simulink library "Ta_Library"  (R2019b)
settings: Solver=VariableStepAuto  StartTime=0.0  StopTime=10.0  RelTol=1e-3
undefined symbols (not defined in the file): AEBSFunctionLib, StateDelayAbortion, TargetClassification
libraries: Mylibrary x5, simulink x1
(part 1 of 3)
settings Model: Creator=hezhaoyang  LastModifiedBy=86156

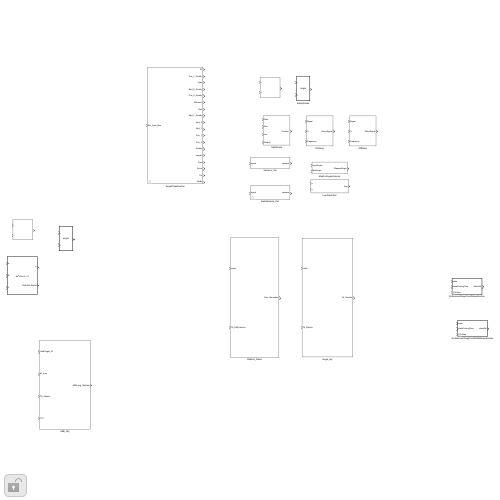
[thumbnail: Simulink's stored preview of the top-level diagram]
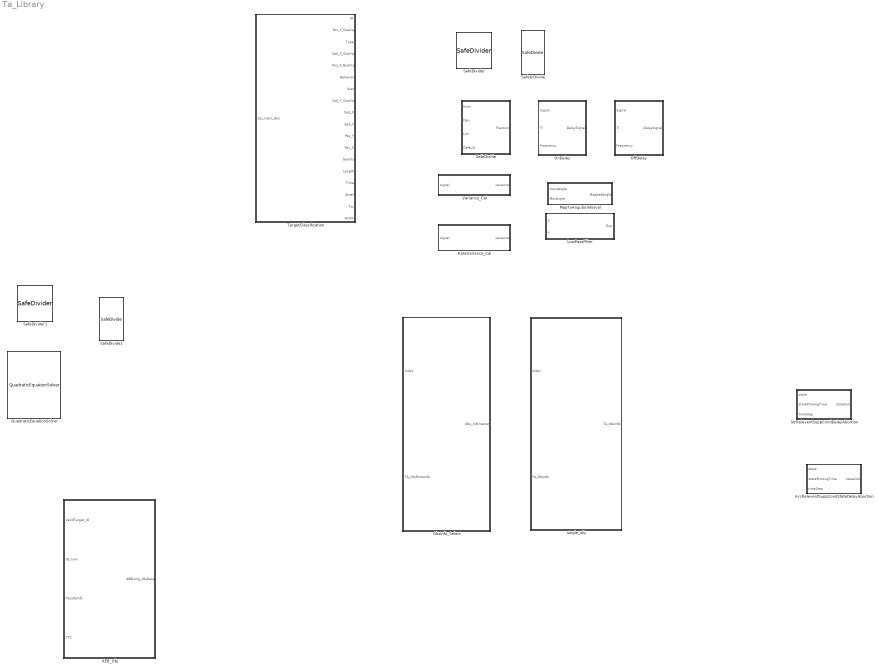
== system Ta_Library ==
  AEB_Obj : Subsystem
  AccReleventSuppCondStateDelayAbortion : Subsystem  AncestorBlock=AEBSFunctionLib/StateDelayAbortion  TreatAsAtomicUnit=on
  LowPassFilter : Subsystem
  MapToAngularInterval : Subsystem
  ObsInfo_Select : Subsystem
  OffDelay : Subsystem
  OnDelay : Subsystem
  QuadraticEquationSolver : Mylibrary/QuadraticEquationSolver  ZeroThreshold=single(1e-2)
  RateVariance_Cal : Subsystem  AncestorBlock=Ta_Library/Variance_Cal
  SafeDivide : Subsystem
  SafeDivide1 : Mylibrary/SafeDivide  DataType=single  DataTypeMax=0  DataTypeMin=0
  SafeDivider : Mylibrary/SafeDivider  SystemSampleTime=-1  Latency=0  AutoFrameSizeCalculation=off
  SafeDivider1 : Mylibrary/SafeDivider  SystemSampleTime=-1  Latency=0  AutoFrameSizeCalculation=off
  SafetyDivide : Mylibrary/SafeDivide  DataType=single  DataTypeMax=0  DataTypeMin=0
  StrReleventSuppCondDelayAbortion : Subsystem  AncestorBlock=AEBSFunctionLib/StateDelayAbortion  TreatAsAtomicUnit=on
  TargetClassification : Subsystem  AncestorBlock=TargetClassification/TargetClassification
  Variance_Cal : Subsystem
  single_obj : Subsystem

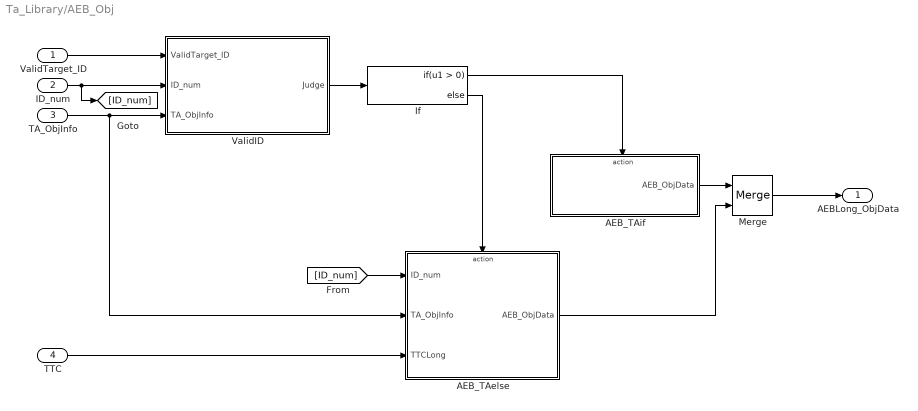
== system Ta_Library/AEB_Obj ==
  ValidTarget_ID : Inport
  ID_num : Inport  Port=2
  TA_ObjInfo : Inport  Port=3
  TTC : Inport  Port=4
  AEB_TAelse : Subsystem  TreatAsAtomicUnit=on
  AEB_TAif : Subsystem  TreatAsAtomicUnit=on
  If : If
  Merge : Merge
  ValidID : Subsystem
  AEBLong_ObjData : Outport
  wires:
  ValidID/1(Judge) -> If/1
  If/1 -> AEB_TAif/Action
  TA_ObjInfo/1 -> AEB_TAelse/2(TA_ObjInfo), ValidID/3(TA_ObjInfo)
  If/2 -> AEB_TAelse/Action
  ID_num/1 -> [ID_num], ValidID/2(ID_num)
  AEB_TAif/1(AEB_ObjData) -> Merge/1
  AEB_TAelse/1(AEB_ObjData) -> Merge/2
  Merge/1 -> AEBLong_ObjData/1
  ValidTarget_ID/1 -> ValidID/1(ValidTarget_ID)
  [ID_num] -> AEB_TAelse/1(ID_num)
  TTC/1 -> AEB_TAelse/3(TTCLong)

== system Ta_Library/AccReleventSuppCondStateDelayAbortion ==
  state : Inport
  stateProlongTime : Inport  Port=2
  timeStep : Inport  Port=3
  StateDelayAbortion : Stateflow chart  TreatAsAtomicUnit=on
  Terminator : Terminator
  Unit Delay : UnitDelay  SampleTime=-1  HasFrameUpgradeWarning=on
  stateOut : Outport
  wires:
  state/1 -> Unit Delay/1, StateDelayAbortion/1(state)
  Unit Delay/1 -> StateDelayAbortion/2(stateK1)
  stateProlongTime/1 -> StateDelayAbortion/3(stateProlongationTime)
  timeStep/1 -> StateDelayAbortion/4(Ts)
  StateDelayAbortion/1(timeSinceLastState) -> Terminator/1
  StateDelayAbortion/2(stateOut) -> stateOut/1

== system Ta_Library/LowPassFilter ==
  a : Inport
  u : Inport  Port=2
  Add3 : Sum
  Delay1 : Delay  DelayLength=1
  Product1 : Product
  Subtract : Sum  Inputs=+-
  Exp : Outport  VectorParamsAs1DForOutWhenUnconnected=off
  wires:
  a/1 -> Product1/1
  Add3/1 -> Delay1/1, Exp/1
  Product1/1 -> Add3/1
  Delay1/1 -> Subtract/2, Add3/2
  Subtract/1 -> Product1/2
  u/1 -> Subtract/1

== system Ta_Library/MapToAngularInterval ==
  note: Map the input angle to an interval between [-MaxAngle, MaxAngle].
  InputAngle : Inport
  MaxAngle : Inport  Port=2
  Gain_1 : Gain  Gain=2  OutDataTypeStr=single
  Modulus : Math  Operator=mod  SignedPower=on  SaturateOnIntegerOverflow=on
  Subtract_1 : Sum  Inputs=-+  OutDataTypeStr=single
  Subtract_2 : Sum  Inputs=+-  OutDataTypeStr=single
  MappedAngle : Outport
  wires:
  [MaxAngle] -> Subtract_2/1
  Gain_1/1 -> Modulus/2
  MaxAngle/1 -> [MaxAngle], Subtract_1/2, Gain_1/1  "MaxAngle"
  InputAngle/1 -> Subtract_1/1  "InputAngle"
  Subtract_1/1 -> Modulus/1
  Modulus/1 -> Subtract_2/2
  Subtract_2/1 -> MappedAngle/1  "MappedAngle"

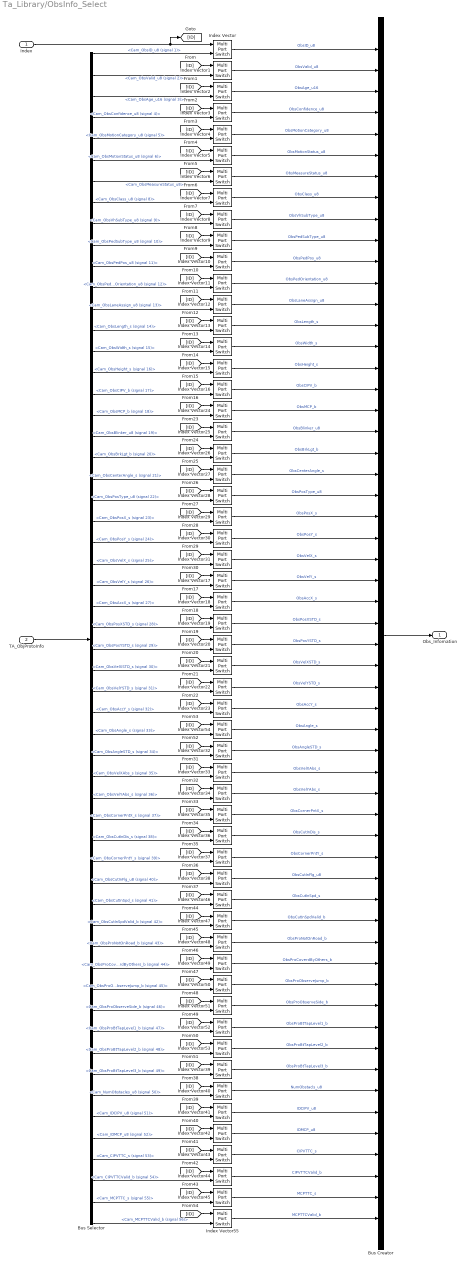
== system Ta_Library/ObsInfo_Select ==
  Index : Inport
  TA_ObjProtoInfo : Inport  Port=2
  Bus Creator : BusCreator  Inputs=56
  Bus Selector : BusSelector  OutputSignals=Cam_ObsID_u8 (signal 1),Cam_ObsValid_u8 (signal 2),Cam_ObsAge_u16 (signal 3),Cam_ObsConfidence_u8 (signal 4),Cam_ObsMotionCategory_u8 (signal 5),Cam_ObsMotionStatus_u8 (signal 6),Cam_ObsMeasureStatus_u8,Cam_ObsClass_u8 (signal 8),Cam_ObsVhSubType_u8 (signal 9),Cam_ObsPedSubType_u8 (signal 10),Cam_ObsPedPos_u8 (signal 11),Cam_ObsPedOrientation_u8 (signal 12),Cam_ObsLaneAssign_u8 (signal 13),Cam_ObsLength_s (signal 14),Cam_ObsWidth_s (signal 15),Cam_ObsHeight_s (signal 16),Cam_ObsCIPV_b (signal 17),Cam_ObsMCP_b (signal 18),Cam_ObsBlinker_u8 (signal 19),Cam_ObsBrkLgt_b (signal 20),Cam_ObsCenterAngle_s (signal 21),Cam_ObsPosType_u8 (signal 22),Cam_ObsPosX_s (signal 23),Cam_ObsPosY_s (signal 24),Cam_ObsVelX_s (signal 25),Cam_ObsVelY_s (signal 26),Cam_ObsAccX_s (signal 27),Cam_ObsPosXSTD_s (signal 28),Cam_ObsPosYSTD_s (signal 29),Cam_ObsVelXSTD_s (signal 30),Cam_ObsVelYSTD_s (signal 31),Cam_ObsAccY_s (signal 32),Cam_ObsAngle_s (signal 33),Cam_ObsAngleSTD_s (signal 34),Cam_ObsVelXAbs_s (signal 35),Cam_ObsVelYAbs_s (signal 36),Cam_ObsCornerPntX_s (signal 37),Cam_ObsCutInDis_s (signal 38),Cam_ObsCornerPntY_s (signal 39),Cam_ObsCutInFlg_u8 (signal 40),Cam_ObsCutInSpd_s (signal 41),Cam_ObsCutInSpdValid_b (signal 42),Cam_ObsProNotOnRoad_b (signal 43),Cam_ObsProCoverdByOthers_b (signal 44),Cam_ObsProObserveJump_b (signal 45),Cam_ObsProObserveSide_b (signal 46),Cam_ObsProBtTapLevel1_b (signal 47),Cam_ObsProBtTapLevel2_b (signal 48),Cam_ObsProBtTapLevel3_b (signal 49),Cam_NumObstacles_u8 (signal 50),Cam_IDCIPV_u8 (signal 51),Cam_IDMCP_u8 (signal 52),Cam_CIPVTTC_s (signal 53),Cam_CIPVTTCValid_b (signal 54),Cam_MCPTTC_s (signal 55),Cam_MCPTTCValid_b (signal 56)
  Index Vector{,1..55} (56 alike) : MultiPortSwitch  Inputs=1
  Obs_Infomation : Outport
  wires:
  TA_ObjProtoInfo/1 -> Bus Selector/1
  Bus Selector/1 -> Index Vector/2  "<Cam_ObsID_u8 (signal 1)>"
  Index/1 -> [ID], Index Vector/1
  [ID] -> Index Vector1/1
  Bus Selector/2 -> Index Vector1/2  "<Cam_ObsValid_u8 (signal 2)>"
  Bus Selector/3 -> Index Vector2/2  "<Cam_ObsAge_u16 (signal 3)>"
  [ID] -> Index Vector2/1
  [ID] -> Index Vector4/1
  Bus Selector/5 -> Index Vector4/2  "<Cam_ObsMotionCategory_u8 (signal 5)>"
  Bus Selector/4 -> Index Vector3/2  "<Cam_ObsConfidence_u8 (signal 4)>"
  [ID] -> Index Vector3/1
  [ID] -> Index Vector7/1
  Bus Selector/8 -> Index Vector7/2  "<Cam_ObsClass_u8 (signal 8)>"
  Bus Selector/9 -> Index Vector8/2  "<Cam_ObsVhSubType_u8 (signal 9)>"
  [ID] -> Index Vector8/1
  [ID] -> Index Vector6/1
  Bus Selector/7 -> Index Vector6/2  "<Cam_ObsMeasureStatus_u8>"
  Bus Selector/6 -> Index Vector5/2  "<Cam_ObsMotionStatus_u8 (signal 6)>"
  [ID] -> Index Vector5/1
  [ID] -> Index Vector13/1
  Bus Selector/14 -> Index Vector13/2  "<Cam_ObsLength_s (signal 14)>"
  Bus Selector/15 -> Index Vector14/2  "<Cam_ObsWidth_s (signal 15)>"
  [ID] -> Index Vector14/1
  [ID] -> Index Vector16/1
  Bus Selector/16 -> Index Vector15/2  "<Cam_ObsHeight_s (signal 16)>"
  [ID] -> Index Vector15/1
  [ID] -> Index Vector11/1
  Bus Selector/12 -> Index Vector11/2  "<Cam_ObsPedOrientation_u8 (signal 12)>"
  Bus Selector/13 -> Index Vector12/2  "<Cam_ObsLaneAssign_u8 (signal 13)>"
  [ID] -> Index Vector12/1
  [ID] -> Index Vector10/1
  Bus Selector/11 -> Index Vector10/2  "<Cam_ObsPedPos_u8 (signal 11)>"
  Bus Selector/10 -> Index Vector9/2  "<Cam_ObsPedSubType_u8 (signal 10)>"
  [ID] -> Index Vector9/1
  Bus Selector/17 -> Index Vector16/2  "<Cam_ObsCIPV_b (signal 17)>"
  Bus Selector/32 -> Index Vector23/2  "<Cam_ObsAccY_s (signal 32)>"
  [ID] -> Index Vector31/1
  Bus Selector/25 -> Index Vector31/2  "<Cam_ObsVelX_s (signal 25)>"
  Bus Selector/26 -> Index Vector17/2  "<Cam_ObsVelY_s (signal 26)>"
  [ID] -> Index Vector17/1
  [ID] -> Index Vector19/1
  Bus Selector/28 -> Index Vector19/2  "<Cam_ObsPosXSTD_s (signal 28)>"
  Bus Selector/27 -> Index Vector18/2  "<Cam_ObsAccX_s (signal 27)>"
  [ID] -> Index Vector18/1
  [ID] -> Index Vector22/1
  Bus Selector/31 -> Index Vector22/2  "<Cam_ObsVelYSTD_s (signal 31)>"
  [ID] -> Index Vector23/1
  [ID] -> Index Vector21/1
  Bus Selector/30 -> Index Vector21/2  "<Cam_ObsVelXSTD_s (signal 30)>"
  Bus Selector/29 -> Index Vector20/2  "<Cam_ObsPosYSTD_s (signal 29)>"
  [ID] -> Index Vector20/1
  [ID] -> Index Vector27/1
  Bus Selector/21 -> Index Vector27/2  "<Cam_ObsCenterAngle_s (signal 21)>"
  Bus Selector/22 -> Index Vector28/2  "<Cam_ObsPosType_u8 (signal 22)>"
  [ID] -> Index Vector28/1
  [ID] -> Index Vector30/1
  Bus Selector/24 -> Index Vector30/2  "<Cam_ObsPosY_s (signal 24)>"
  Bus Selector/23 -> Index Vector29/2  "<Cam_ObsPosX_s (signal 23)>"
  [ID] -> Index Vector29/1
  [ID] -> Index Vector25/1
  Bus Selector/19 -> Index Vector25/2  "<Cam_ObsBlinker_u8 (signal 19)>"
  Bus Selector/20 -> Index Vector26/2  "<Cam_ObsBrkLgt_b (signal 20)>"
  [ID] -> Index Vector26/1
  [ID] -> Index Vector24/1
  Bus Selector/18 -> Index Vector24/2  "<Cam_ObsMCP_b (signal 18)>"
  Bus Selector/41 -> Index Vector46/2  "<Cam_ObsCutInSpd_s (signal 41)>"
  [ID] -> Index Vector46/1
  [ID] -> Index Vector48/1
  Bus Selector/43 -> Index Vector48/2  "<Cam_ObsProNotOnRoad_b (signal 43)>"
  Bus Selector/42 -> Index Vector47/2  "<Cam_ObsCutInSpdValid_b (signal 42)>"
  [ID] -> Index Vector47/1
  [ID] -> Index Vector51/1
  Bus Selector/46 -> Index Vector51/2  "<Cam_ObsProObserveSide_b (signal 46)>"
  Bus Selector/47 -> Index Vector52/2  "<Cam_ObsProBtTapLevel1_b (signal 47)>"
  [ID] -> Index Vector52/1
  [ID] -> Index Vector50/1
  Bus Selector/45 -> Index Vector50/2  "<Cam_ObsProObserveJump_b (signal 45)>"
  Bus Selector/44 -> Index Vector49/2  "<Cam_ObsProCoverdByOthers_b (signal 44)>"
  [ID] -> Index Vector49/1
  [ID] -> Index Vector42/1
  Bus Selector/52 -> Index Vector42/2  "<Cam_IDMCP_u8 (signal 52)>"
  Bus Selector/53 -> Index Vector43/2  "<Cam_CIPVTTC_s (signal 53)>"
  [ID] -> Index Vector43/1
  [ID] -> Index Vector45/1
  Bus Selector/54 -> Index Vector44/2  "<Cam_CIPVTTCValid_b (signal 54)>"
  [ID] -> Index Vector44/1
  [ID] -> Index Vector40/1
  Bus Selector/50 -> Index Vector40/2  "<Cam_NumObstacles_u8 (signal 50)>"
  Bus Selector/51 -> Index Vector41/2  "<Cam_IDCIPV_u8 (signal 51)>"
  [ID] -> Index Vector41/1
  [ID] -> Index Vector39/1
  Bus Selector/49 -> Index Vector39/2  "<Cam_ObsProBtTapLevel3_b (signal 49)>"
  Bus Selector/48 -> Index Vector53/2  "<Cam_ObsProBtTapLevel2_b (signal 48)>"
  [ID] -> Index Vector53/1
  Bus Selector/55 -> Index Vector45/2  "<Cam_MCPTTC_s (signal 55)>"
  Bus Selector/40 -> Index Vector38/2  "<Cam_ObsCutInFlg_u8 (signal 40)>"
  Bus Selector/33 -> Index Vector54/2  "<Cam_ObsAngle_s (signal 33)>"
  Bus Selector/34 -> Index Vector32/2  "<Cam_ObsAngleSTD_s (signal 34)>"
  [ID] -> Index Vector32/1
  [ID] -> Index Vector34/1
  Bus Selector/36 -> Index Vector34/2  "<Cam_ObsVelYAbs_s (signal 36)>"
  Bus Selector/35 -> Index Vector33/2  "<Cam_ObsVelXAbs_s (signal 35)>"
  [ID] -> Index Vector33/1
  [ID] -> Index Vector37/1
  Bus Selector/39 -> Index Vector37/2  "<Cam_ObsCornerPntY_s (signal 39)>"
  [ID] -> Index Vector38/1
  [ID] -> Index Vector36/1
  Bus Selector/38 -> Index Vector36/2  "<Cam_ObsCutInDis_s (signal 38)>"
  Bus Selector/37 -> Index Vector35/2  "<Cam_ObsCornerPntX_s (signal 37)>"
  [ID] -> Index Vector35/1
  [ID] -> Index Vector54/1
  Bus Selector/56 -> Index Vector55/2  "<Cam_MCPTTCValid_b (signal 56)>"
  [ID] -> Index Vector55/1
  Index Vector32/1 -> Bus Creator/34  "ObsAngleSTD_s"
  Index Vector33/1 -> Bus Creator/35  "ObsVelXAbs_s"
  Index Vector54/1 -> Bus Creator/33  "ObsAngle_s"
  Index Vector34/1 -> Bus Creator/36  "ObsVelYAbs_s"
  Index Vector23/1 -> Bus Creator/32  "ObsAccY_s"
  Index Vector35/1 -> Bus Creator/37  "ObsCornerPntX_s"
  Index Vector22/1 -> Bus Creator/31  "ObsVelYSTD_s"
  Index Vector36/1 -> Bus Creator/38  "ObsCutInDis_s"
  Index Vector21/1 -> Bus Creator/30  "ObsVelXSTD_s"
  Index Vector37/1 -> Bus Creator/39  "ObsCornerPntY_s"
  Index Vector20/1 -> Bus Creator/29  "ObsPosYSTD_s"
  Index Vector38/1 -> Bus Creator/40  "ObsCutInFlg_u8"
  Index Vector19/1 -> Bus Creator/28  "ObsPosXSTD_s"
  Index Vector46/1 -> Bus Creator/41  "ObsCutInSpd_s"
  Index Vector18/1 -> Bus Creator/27  "ObsAccX_s"
  Index Vector47/1 -> Bus Creator/42  "ObsCutInSpdValid_b"
  Index Vector17/1 -> Bus Creator/26  "ObsVelY_s"
  Index Vector48/1 -> Bus Creator/43  "ObsProNotOnRoad_b"
  Index Vector31/1 -> Bus Creator/25  "ObsVelX_s"
  Index Vector49/1 -> Bus Creator/44  "ObsProCoverdByOthers_b"
  Index Vector30/1 -> Bus Creator/24  "ObsPosY_s"
  Index Vector50/1 -> Bus Creator/45  "ObsProObserveJump_b"
  Index Vector29/1 -> Bus Creator/23  "ObsPosX_s"
  Index Vector51/1 -> Bus Creator/46  "ObsProObserveSide_b"
  Index Vector28/1 -> Bus Creator/22  "ObsPosType_u8"
  Index Vector52/1 -> Bus Creator/47  "ObsProBtTapLevel1_b"
  Index Vector27/1 -> Bus Creator/21  "ObsCenterAngle_s"
  Index Vector53/1 -> Bus Creator/48  "ObsProBtTapLevel2_b"
  Index Vector26/1 -> Bus Creator/20  "ObsBrkLgt_b"
  Index Vector39/1 -> Bus Creator/49  "ObsProBtTapLevel3_b"
  Index Vector25/1 -> Bus Creator/19  "ObsBlinker_u8"
  Index Vector40/1 -> Bus Creator/50  "NumObstacls_u8"
  Index Vector24/1 -> Bus Creator/18  "ObsMCP_b"
  Index Vector41/1 -> Bus Creator/51  "IDCIPV_u8"
  Index Vector16/1 -> Bus Creator/17  "ObsCIPV_b"
  Index Vector42/1 -> Bus Creator/52  "IDMCP_u8"
  Index Vector15/1 -> Bus Creator/16  "ObsHeight_s"
  Index Vector43/1 -> Bus Creator/53  "CIPVTTC_s"
  Index Vector14/1 -> Bus Creator/15  "ObsWidth_s"
  Index Vector44/1 -> Bus Creator/54  "CIPVTTCValid_b"
  Index Vector13/1 -> Bus Creator/14  "ObsLength_s"
  Index Vector45/1 -> Bus Creator/55  "MCPTTC_s"
  Index Vector12/1 -> Bus Creator/13  "ObsLaneAssign_u8"
  Index Vector55/1 -> Bus Creator/56  "MCPTTCValid_b"
  Index Vector11/1 -> Bus Creator/12  "ObsPedOrientation_u8"
  Index Vector10/1 -> Bus Creator/11  "ObsPedPos_u8"
  Index Vector9/1 -> Bus Creator/10  "ObsPedSubType_u8"
  Index Vector8/1 -> Bus Creator/9  "ObsVhSubType_u8"
  Index Vector7/1 -> Bus Creator/8  "ObsClass_u8"
  Index Vector6/1 -> Bus Creator/7  "ObsMeasureStatus_u8"
  Index Vector5/1 -> Bus Creator/6  "ObsMotionStatus_u8"
  Index Vector4/1 -> Bus Creator/5  "ObsMotionCategory_u8"
  Index Vector3/1 -> Bus Creator/4  "ObsConfidence_u8"
  Index Vector2/1 -> Bus Creator/3  "ObsAge_u16"
  Index Vector1/1 -> Bus Creator/2  "ObsValid_u8"
  Index Vector/1 -> Bus Creator/1  "ObsID_u8"
  Bus Creator/1 -> Obs_Infomation/1

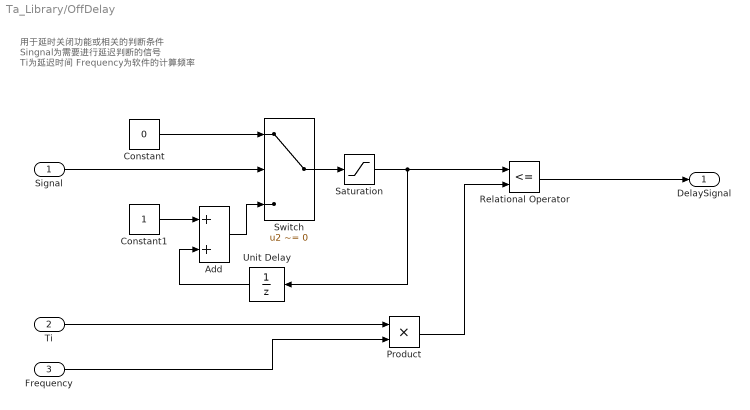
== system Ta_Library/OffDelay ==
  note: 用于延时关闭功能或相关的判断条件
      | Singnal为需要进行延迟判断的信号
      | Ti为延迟时间
      | Frequency为软件的计算频率
  Signal : Inport
  Ti : Inport  Port=2
  Frequency : Inport  Port=3
  Add : Sum
  Constant : Constant  Value=0  OutDataTypeStr=single
  Constant1 : Constant  OutDataTypeStr=single
  Product : Product
  Relational Operator : RelationalOperator  Operator=<=  OutDataTypeStr=boolean  RndMeth=Simplest
  Saturation : Saturate  UpperLimit=1000  LowerLimit=0
  Switch : Switch  Criteria=u2 ~= 0
  Unit Delay : UnitDelay  SampleTime=-1  HasFrameUpgradeWarning=on
  DelaySignal : Outport
  wires:
  Signal/1 -> Switch/2
  Ti/1 -> Product/1
  Constant1/1 -> Add/1
  Unit Delay/1 -> Add/2
  Switch/1 -> Saturation/1
  Constant/1 -> Switch/1
  Relational Operator/1 -> DelaySignal/1
  Frequency/1 -> Product/2
  Product/1 -> Relational Operator/2
  Add/1 -> Switch/3
  Saturation/1 -> Relational Operator/1, Unit Delay/1

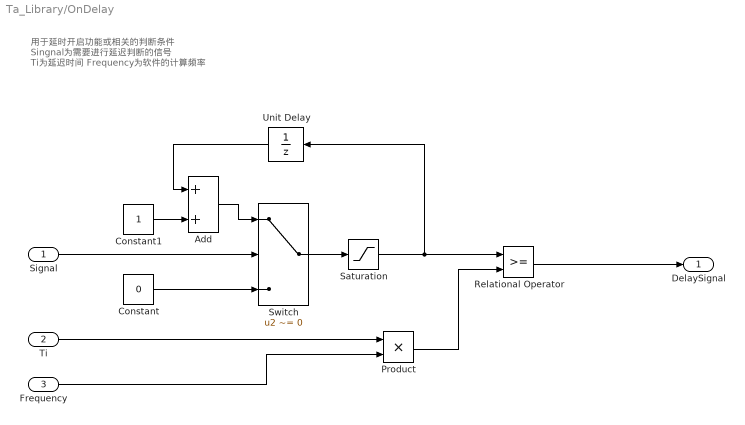
== system Ta_Library/OnDelay ==
  note: 用于延时开启功能或相关的判断条件
      | Singnal为需要进行延迟判断的信号
      | Ti为延迟时间
      | Frequency为软件的计算频率
  Signal : Inport
  Ti : Inport  Port=2
  Frequency : Inport  Port=3
  Add : Sum
  Constant : Constant  Value=0  OutDataTypeStr=single
  Constant1 : Constant  OutDataTypeStr=single
  Product : Product
  Relational Operator : RelationalOperator  OutDataTypeStr=boolean  RndMeth=Simplest
  Saturation : Saturate  UpperLimit=1000  LowerLimit=0
  Switch : Switch  Criteria=u2 ~= 0
  Unit Delay : UnitDelay  SampleTime=-1  HasFrameUpgradeWarning=on
  DelaySignal : Outport
  wires:
  Product/1 -> Relational Operator/2
  Switch/1 -> Saturation/1
  Ti/1 -> Product/1
  Signal/1 -> Switch/2
  Relational Operator/1 -> DelaySignal/1
  Frequency/1 -> Product/2
  Add/1 -> Switch/1
  Constant/1 -> Switch/3
  Constant1/1 -> Add/2
  Unit Delay/1 -> Add/1
  Saturation/1 -> Relational Operator/1, Unit Delay/1

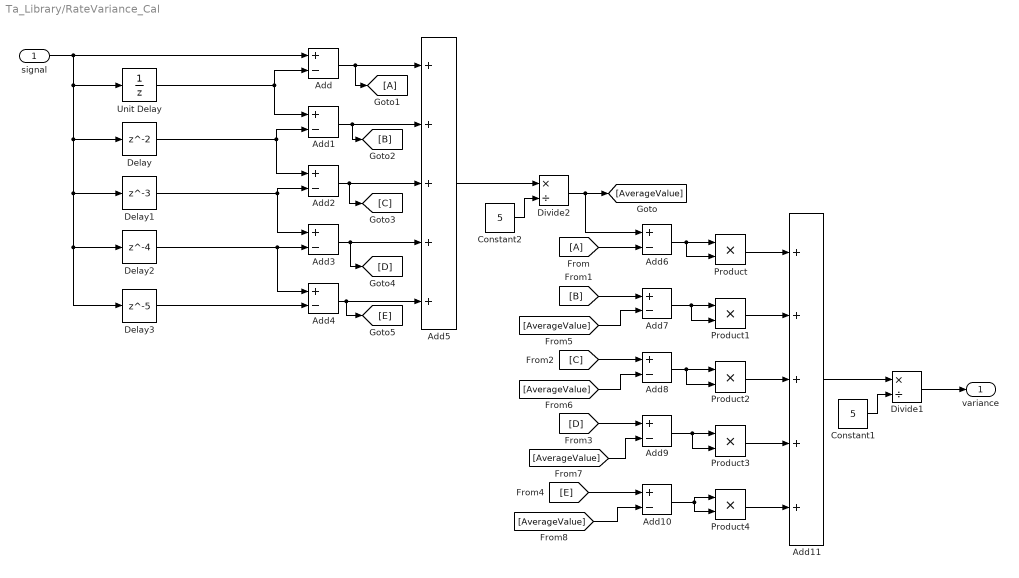
== system Ta_Library/RateVariance_Cal ==
  signal : Inport
  Add{,1..4,6..10} (10 alike) : Sum  Inputs=+-
  Add11 : Sum  Inputs=+++++
  Add5 : Sum  Inputs=+++++
  Constant1 : Constant  Value=5  OutDataTypeStr=single
  Constant2 : Constant  Value=5  OutDataTypeStr=single
  Delay : Delay
  Delay1 : Delay  DelayLength=3
  Delay2 : Delay  DelayLength=4
  Delay3 : Delay  DelayLength=5
  Divide1 : Product  Inputs=*/
  Divide2 : Product  Inputs=*/
  Product{,1..4} (5 alike) : Product
  Unit Delay : UnitDelay  SampleTime=-1  HasFrameUpgradeWarning=on
  variance : Outport
  wires:
  Divide1/1 -> variance/1
  Constant1/1 -> Divide1/2
  Unit Delay/1 -> Add1/1, Add/2
  Delay/1 -> Add2/1, Add1/2
  Delay1/1 -> Add3/1, Add2/2
  Delay3/1 -> Add4/2
  Delay2/1 -> Add4/1, Add3/2
  signal/1 -> Delay3/1, Delay2/1, Delay1/1, Delay/1, Unit Delay/1, Add/1
  Add/1 -> [A], Add5/1
  Add1/1 -> [B], Add5/2
  Add2/1 -> [C], Add5/3
  Add3/1 -> [D], Add5/4
  Add4/1 -> [E], Add5/5
  Add5/1 -> Divide2/1
  Constant2/1 -> Divide2/2
  Divide2/1 -> Add6/1, [AverageValue]
  [A] -> Add6/2
  Add6/1 -> Product/2, Product/1
  [B] -> Add7/1
  [AverageValue] -> Add7/2
  Add7/1 -> Product1/2, Product1/1
  [C] -> Add8/1
  [AverageValue] -> Add8/2
  Add8/1 -> Product2/2, Product2/1
  [D] -> Add9/1
  [AverageValue] -> Add9/2
  Add9/1 -> Product3/2, Product3/1
  [E] -> Add10/1
  [AverageValue] -> Add10/2
  Add10/1 -> Product4/1, Product4/2
  Product/1 -> Add11/1
  Product1/1 -> Add11/2
  Product2/1 -> Add11/3
  Product3/1 -> Add11/4
  Product4/1 -> Add11/5
  Add11/1 -> Divide1/1

== system Ta_Library/SafeDivide ==
  note: 此模块用于防止除零或被除数过小导致的溢出，Num为被除数，Den为除数，Lim为除数限制，Default是出现除零默认的除数，按照不同情况进行设置
  Num : Inport
  Den : Inport  Port=2
  Lim : Inport  Port=3
  Default : Inport  Port=4
  Abs : Abs
  Divide : Product  Inputs=*/
  Relational Operator : RelationalOperator  Operator=<=  OutDataTypeStr=boolean  RndMeth=Simplest
  Switch : Switch  Criteria=u2 ~= 0
  "Fraction " : Outport
  wires:
  Relational Operator/1 -> Switch/2
  Divide/1 -> "Fraction "/1
  Den/1 -> Switch/1, Abs/1
  Switch/1 -> Divide/2
  Num/1 -> Divide/1
  Lim/1 -> Relational Operator/2
  Default/1 -> Switch/3
  Abs/1 -> Relational Operator/1

== system Ta_Library/StrReleventSuppCondDelayAbortion ==
  state : Inport
  stateProlongTime : Inport  Port=2
  timeStep : Inport  Port=3
  StateDelayAbortion : Stateflow chart  TreatAsAtomicUnit=on
  Terminator : Terminator
  Unit Delay : UnitDelay  SampleTime=-1  HasFrameUpgradeWarning=on
  stateOut : Outport
  wires:
  state/1 -> Unit Delay/1, StateDelayAbortion/1(state)
  Unit Delay/1 -> StateDelayAbortion/2(stateK1)
  stateProlongTime/1 -> StateDelayAbortion/3(stateProlongationTime)
  timeStep/1 -> StateDelayAbortion/4(Ts)
  StateDelayAbortion/1(timeSinceLastState) -> Terminator/1
  StateDelayAbortion/2(stateOut) -> stateOut/1
